simulink model "lab05par02"  (R2015a)
settings: Solver=ode45  StartTime=0.0  StopTime=10.0  RelTol=1e-3
settings Model: Creator=dg  LastModifiedBy=dg

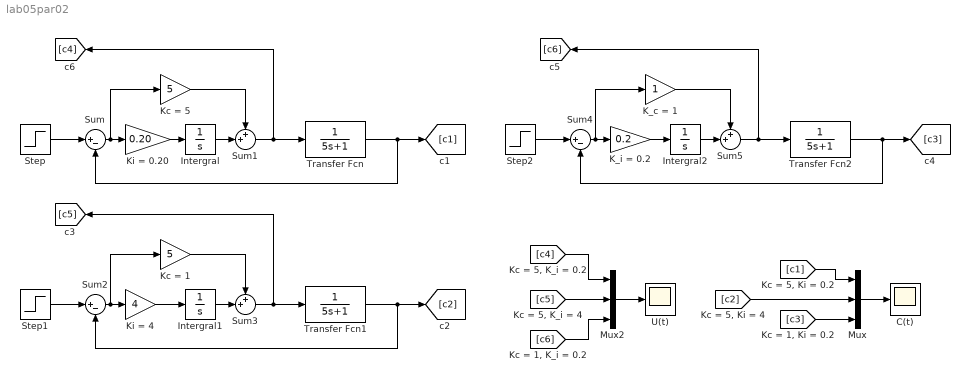
== system lab05par02 ==
  C(t) : Scope
  Intergral : Integrator
  Intergral1 : Integrator
  Intergral2 : Integrator
  K_c = 1 : Gain
  K_i = 0.2 : Gain  Gain=0.2
  Kc = 1 : Gain  Gain=5
  Kc = 5 : Gain  Gain=5
  "Ki = 0.20 " : Gain  Gain=0.20
  Ki = 4 : Gain  Gain=4
  Mux : Mux  Inputs=3
  Mux2 : Mux  Inputs=3
  Step : Step  Time=0  SampleTime=0
  Step1 : Step  Time=0  SampleTime=0
  Step2 : Step  Time=0  SampleTime=0
  Sum : Sum  Inputs=|+-
  Sum1 : Sum  Inputs=++|
  Sum2 : Sum  Inputs=|+-
  Sum3 : Sum  Inputs=++|
  Sum4 : Sum  Inputs=|+-
  Sum5 : Sum  Inputs=++|
  Transfer Fcn : TransferFcn  Denominator=[5 1]
  Transfer Fcn1 : TransferFcn  Denominator=[5 1]
  Transfer Fcn2 : TransferFcn  Denominator=[5 1]
  U(t) : Scope
  wires:
  Step/1 -> Sum/1
  Sum/1 -> Kc = 5/1, "Ki = 0.20 "/1
  "Ki = 0.20 "/1 -> Intergral/1
  Transfer Fcn/1 -> Sum/2, [c1]
  Kc = 5/1 -> Sum1/1
  Intergral/1 -> Sum1/2
  Sum1/1 -> [c4], Transfer Fcn/1
  Step1/1 -> Sum2/1
  Sum2/1 -> Kc = 1/1, Ki = 4/1
  Ki = 4/1 -> Intergral1/1
  Transfer Fcn1/1 -> Sum2/2, [c2]
  Kc = 1/1 -> Sum3/1
  Intergral1/1 -> Sum3/2
  Sum3/1 -> [c5], Transfer Fcn1/1
  Step2/1 -> Sum4/1
  Sum4/1 -> K_c = 1/1, K_i = 0.2/1
  K_i = 0.2/1 -> Intergral2/1
  Transfer Fcn2/1 -> Sum4/2, [c3]
  K_c = 1/1 -> Sum5/1
  Intergral2/1 -> Sum5/2
  Sum5/1 -> [c6], Transfer Fcn2/1
  Mux/1 -> C(t)/1
  [c1] -> Mux/1
  [c2] -> Mux/2
  [c3] -> Mux/3
  Mux2/1 -> U(t)/1
  [c4] -> Mux2/1
  [c6] -> Mux2/3
  [c5] -> Mux2/2
